simulink model "Quad_Nonlinear_LQR"  (R2020a)
settings: Solver=ode4  StartTime=0.0  StopTime=10.0  FixedStep=.02  RelTol=1e-3
InitFcn:
  | init
undefined symbols (not defined in the file or in its folder): b, d_cg, g, h_cg, J_yy, m2, m_tot, magnitude, miu_k, q1, q2, r_y
settings Model: Creator=Ali  LastModifiedBy=Ali

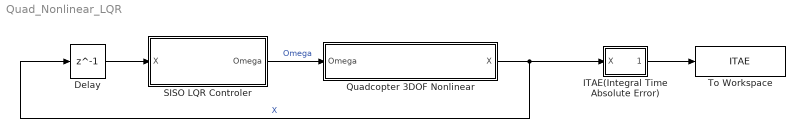
== system Quad_Nonlinear_LQR ==
  Delay : Delay  DelayLength=1
  ITAE(Integral Time Absolute Error) : Subsystem
  Quadcopter 3DOF Nonlinear : Subsystem  TreatAsAtomicUnit=on
  SISO LQR Controler : Subsystem
  To Workspace : ToWorkspace  VariableName=ITAE  SaveFormat=Timeseries  SampleTime=-1
  wires:
  SISO LQR Controler/1(Omega) -> Quadcopter 3DOF Nonlinear/1(Omega)  "Omega"
  Delay/1 -> SISO LQR Controler/1(X)
  Quadcopter 3DOF Nonlinear/1(X) -> ITAE(Integral Time Absolute Error)/1(X), Delay/1  "X"
  ITAE(Integral Time Absolute Error)/1(ITAE) -> To Workspace/1

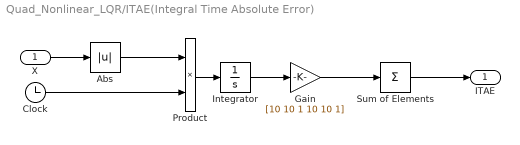
== system Quad_Nonlinear_LQR/ITAE(Integral Time Absolute Error) ==
  X : Inport
  Abs : Abs
  Clock : Clock
  Gain : Gain  Gain=[10 10 1 10 10 1]
  Integrator : Integrator
  Product : Product
  Sum of Elements : Sum  Inputs=+
  ITAE : Outport
  wires:
  Product/1 -> Integrator/1
  Integrator/1 -> Gain/1
  Clock/1 -> Product/2
  Sum of Elements/1 -> ITAE/1
  Abs/1 -> Product/1
  X/1 -> Abs/1
  Gain/1 -> Sum of Elements/1

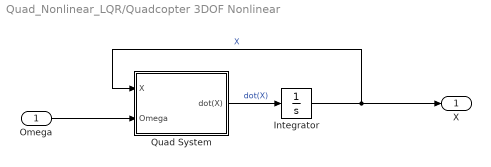
== system Quad_Nonlinear_LQR/Quadcopter 3DOF Nonlinear ==
  Omega : Inport
  Integrator : Integrator  InitialCondition=[-40*pi/180 4*pi/180]
  Quad System : Subsystem
  X : Outport
  wires:
  Integrator/1 -> Quad System/1(X), X/1  "X"
  Quad System/1(dot(X)) -> Integrator/1  "dot(X)"
  Omega/1 -> Quad System/2(Omega)

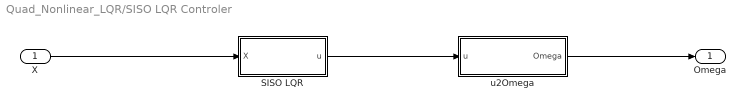
== system Quad_Nonlinear_LQR/SISO LQR Controler ==
  X : Inport
  SISO LQR : Subsystem
  u2Omega : Subsystem
  Omega : Outport
  wires:
  X/1 -> SISO LQR/1(X)
  SISO LQR/1(u) -> u2Omega/1(u)
  u2Omega/1(Omega) -> Omega/1

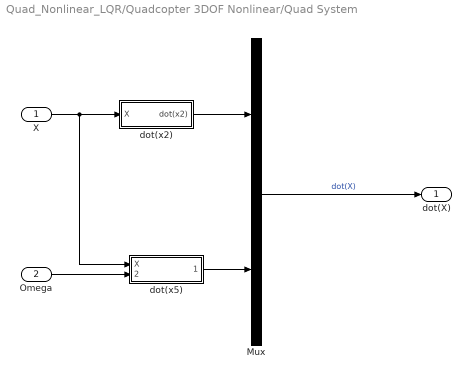
== system Quad_Nonlinear_LQR/Quadcopter 3DOF Nonlinear/Quad System ==
  X : Inport
  Omega : Inport  Port=2
  Mux : Mux  Inputs=2
  dot(x2) : Subsystem
  dot(x5) : Subsystem
  dot(X) : Outport
  wires:
  Mux/1 -> dot(X)/1  "dot(X)"
  dot(x2)/1(dot(x2)) -> Mux/1
  dot(x5)/1(dot(x5)) -> Mux/2
  X/1 -> dot(x5)/1(X), dot(x2)/1(X)
  Omega/1 -> dot(x5)/2(Omega)

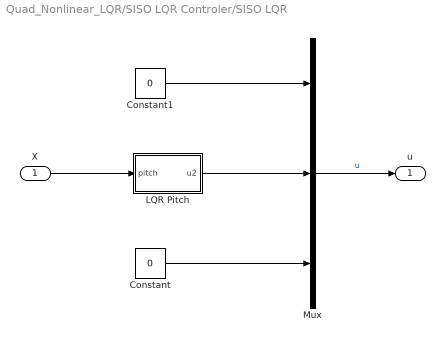
== system Quad_Nonlinear_LQR/SISO LQR Controler/SISO LQR ==
  X : Inport
  Constant : Constant  Value=0
  Constant1 : Constant  Value=0
  LQR Pitch : Subsystem
  Mux : Mux  Inputs=3
  u : Outport
  wires:
  Mux/1 -> u/1  "u"
  Constant1/1 -> Mux/1
  Constant/1 -> Mux/3
  X/1 -> LQR Pitch/1(pitch)
  LQR Pitch/1(u2) -> Mux/2

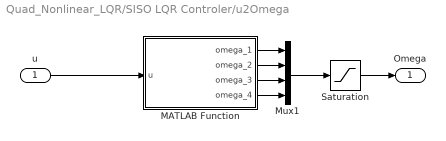
== system Quad_Nonlinear_LQR/SISO LQR Controler/u2Omega ==
  u : Inport
  MATLAB Function : MATLAB Function  TreatAsAtomicUnit=on
  Mux1 : Mux
  Saturation : Saturate  UpperLimit=6000/60*2*pi  LowerLimit=1500/60*2*pi
  Omega : Outport
  wires:
  u/1 -> MATLAB Function/1(u)
  MATLAB Function/3(omega_3) -> Mux1/3
  Mux1/1 -> Saturation/1
  MATLAB Function/1(omega_1) -> Mux1/1
  MATLAB Function/2(omega_2) -> Mux1/2
  MATLAB Function/4(omega_4) -> Mux1/4
  Saturation/1 -> Omega/1

== system Quad_Nonlinear_LQR/Quadcopter 3DOF Nonlinear/Quad System/dot(x2) ==
  X : Inport
  1 : Subsystem
  dot(x2) : Outport
  wires:
  X/1 -> 1/1(X)  "X"
  1/1(x5cos(x1)) -> dot(x2)/1

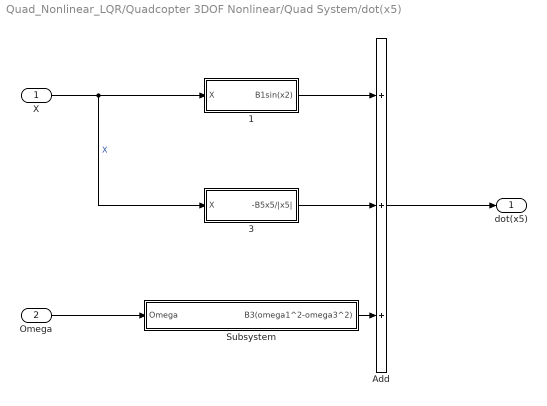
== system Quad_Nonlinear_LQR/Quadcopter 3DOF Nonlinear/Quad System/dot(x5) ==
  X : Inport
  Omega : Inport  Port=2
  1 : Subsystem
  3 : Subsystem
  Add : Sum  Inputs=+++
  Subsystem : Subsystem
  dot(x5) : Outport
  wires:
  X/1 -> 3/1(X), 1/1(X)  "X"
  Omega/1 -> Subsystem/1(Omega)
  Add/1 -> dot(x5)/1
  Subsystem/1(B3(omega1^2-omega3^2)) -> Add/3
  3/1("-B5x5/|x5| ") -> Add/2
  1/1(B1sin(x2)) -> Add/1

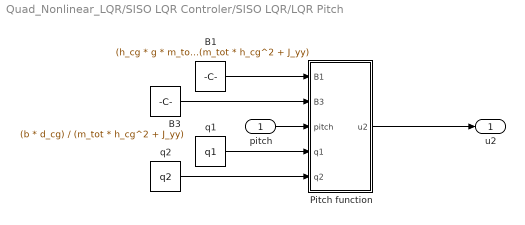
== system Quad_Nonlinear_LQR/SISO LQR Controler/SISO LQR/LQR Pitch ==
  pitch : Inport
  B1 : Constant  Value=(h_cg * g * m_tot) / (m_tot * h_cg^2 + J_yy)
  B3 : Constant  Value=(b * d_cg) / (m_tot * h_cg^2 + J_yy)
  Pitch function : MATLAB Function  TreatAsAtomicUnit=on
  q1 : Constant  Value=q1
  q2 : Constant  Value=q2
  u2 : Outport
  wires:
  Pitch function/1(u2) -> u2/1
  pitch/1 -> Pitch function/3(pitch)
  B1/1 -> Pitch function/1(B1)
  B3/1 -> Pitch function/2(B3)
  q1/1 -> Pitch function/4(q1)
  q2/1 -> Pitch function/5(q2)

== system Quad_Nonlinear_LQR/Quadcopter 3DOF Nonlinear/Quad System/dot(x2)/1 ==
  X : Inport
  Selector : Selector  InputPortWidth=2  IndexOptions=Index vector (dialog)  Indices=[2]  OutputSizes=1
  x5cos(x1) : Outport
  wires:
  X/1 -> Selector/1  "x"
  Selector/1 -> x5cos(x1)/1

== system Quad_Nonlinear_LQR/Quadcopter 3DOF Nonlinear/Quad System/dot(x5)/1 ==
  X : Inport
  Selector : Selector  InputPortWidth=2  IndexOptions=Index vector (dialog)  Indices=[1]  OutputSizes=1
  Subsystem : Subsystem
  B1sin(x2) : Outport
  wires:
  X/1 -> Selector/1  "x"
  Subsystem/1(B1sin(x2)) -> B1sin(x2)/1
  Selector/1 -> Subsystem/1(x2)

== system Quad_Nonlinear_LQR/Quadcopter 3DOF Nonlinear/Quad System/dot(x5)/3 ==
  X : Inport
  Selector : Selector  InputPortWidth=2  IndexOptions=Index vector (dialog)  Indices=[2]  OutputSizes=1
  Subsystem : Subsystem
  "-B5x5/|x5| " : Outport
  wires:
  X/1 -> Selector/1  "x"
  Subsystem/1("-B5x5/|x5| ") -> "-B5x5/|x5| "/1
  Selector/1 -> Subsystem/1(x5)

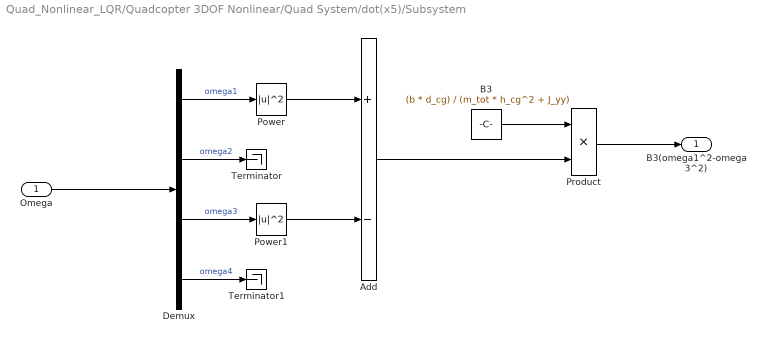
== system Quad_Nonlinear_LQR/Quadcopter 3DOF Nonlinear/Quad System/dot(x5)/Subsystem ==
  Omega : Inport
  Add : Sum  Inputs=+-
  B3 : Constant  Value=(b * d_cg) / (m_tot * h_cg^2 + J_yy)
  Demux : Demux
  Power : Math  Operator=magnitude^2  SaturateOnIntegerOverflow=on
  Power1 : Math  Operator=magnitude^2  SaturateOnIntegerOverflow=on
  Product : Product
  Terminator : Terminator
  Terminator1 : Terminator
  B3(omega1^2-omega3^2) : Outport
  wires:
  Product/1 -> B3(omega1^2-omega3^2)/1
  Power1/1 -> Add/2
  Add/1 -> Product/2
  Power/1 -> Add/1
  B3/1 -> Product/1
  Omega/1 -> Demux/1
  Demux/3 -> Power1/1  "omega3"
  Demux/1 -> Power/1  "omega1"
  Demux/2 -> Terminator/1  "omega2"
  Demux/4 -> Terminator1/1  "omega4"

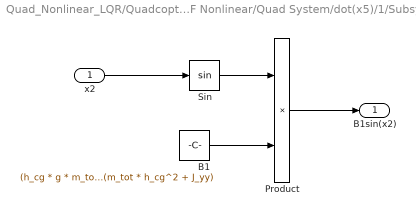
== system Quad_Nonlinear_LQR/Quadcopter 3DOF Nonlinear/Quad System/dot(x5)/1/Subsystem ==
  x2 : Inport
  B1 : Constant  Value=(h_cg * g * m_tot) / (m_tot * h_cg^2 + J_yy)
  Product : Product
  Sin : Trigonometry
  B1sin(x2) : Outport
  wires:
  Product/1 -> B1sin(x2)/1
  x2/1 -> Sin/1
  Sin/1 -> Product/1
  B1/1 -> Product/2

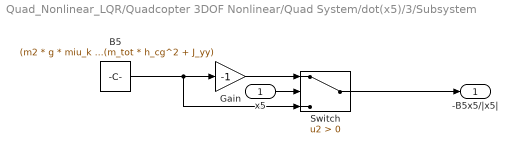
== system Quad_Nonlinear_LQR/Quadcopter 3DOF Nonlinear/Quad System/dot(x5)/3/Subsystem ==
  x5 : Inport
  B5 : Constant  Value=(m2 * g * miu_k * r_y) / (m_tot * h_cg^2 + J_yy)
  Gain : Gain  Gain=-1
  Switch : Switch  Criteria=u2 > Threshold
  "-B5x5/|x5| " : Outport
  wires:
  Switch/1 -> "-B5x5/|x5| "/1
  B5/1 -> Switch/3, Gain/1
  x5/1 -> Switch/2
  Gain/1 -> Switch/1

== matlab function Quad_Nonlinear_LQR/SISO LQR Controler/SISO LQR/LQR Pitch/Pitch function ==
  data: B1 input; B3 input; pitch input; u2 output; q1 input; q2 input
function u2  = fcn(B1, B3, pitch, q1, q2)

x2     = pitch(1);
A22    = 0; %da2dx2
A25    = 1; %da2dx5
A52    = B1 * cos(x2); %da5dx2
A55    = 0; %da5dx5

A      = [A22, A25 ;
          A52, A55];
B      = [0  ;
          B3];
a      = A(2);
b      = B(2);

R      = 1;
R_inv  = R^-1;
K_ans = zeros(2, 2);
% algebraic_riccati = K * A + A' * K - K * B * R^-1 * B' * K + Q;
% first equation q1 + 2*a*k12 - (b^2*k12^2)/R = 0
% Ans1 K12 = -m*(k + (k^2 + Q11)^(1/2))
% Ans2 K12 = -m*(k - (k^2 + Q11)^(1/2))
K12 = zeros(1, 2);
K12(1) = (R*(a + ((R*a^2 + q1*b^2)/R)^(1/2)))/b^2;
K12(2) = (R*(a - ((R*a^2 + q1*b^2)/R)^(1/2)))/b^2;
stable = false; % check stability answer for break code
for i = 1:length(K12)
    % Second equation 2*k12 + q2 - (b^2*k22^2)/R = 0
    % Ans1 K12 =  (2*k12 + q2)^(1/2)/(R^(1/2)*b)
    % Ans2 K12 = -(2*k12 + q2)^(1/2)/(R^(1/2)*b)
    valid22 = [true; true]; % for validation in complex number
    K22 = zeros(1, 2);
    if (2*K12(i) + q2) < 0
        valid22(i) = false;
    end
    if valid22(i)
        K22(1) =  (R^(1/2)*(2*K12(i) + q2)^(1/2))/b;
        K22(2) = -(R^(1/2)*(2*K12(i) + q2)^(1/2))/b;
    else
        continue;
    end
    for j = 1:length(K22)
        % Last equation k11 + a*k22 - (b^2*k12*k22)/R = 0
        % Ans R*k12*k22*b^2 - a*k22
        K11 = (K12(i)*K22(j)*b^2)/R - a*K22(j);
        temp_K = zeros(2, 2);
        temp_K(1, 1) = K11;
        temp_K(1, 2) = K12(i);
        temp_K(2, 1) = K12(i);
        temp_K(2, 2) = K22(j);
        if all(eig(A - B * R^(-1)* B' * temp_K) < 0)
            K_ans = temp_K;
            stable = true;
            break;
        end
    end
    if stable
        break;
    end
end

u2 = -R_inv*B'*K_ans*pitch;

== matlab function Quad_Nonlinear_LQR/SISO LQR Controler/u2Omega/MATLAB Function ==
  data: u input size=3; omega_1 output size=1; omega_2 output size=1; omega_3 output size=1; omega_4 output size=1
function [omega_1, omega_2, omega_3, omega_4] = fcn(u)
u1 = u(1);
u2 = u(2);
u3 = u(3);
% control effort
u4 = ones(1, length(u1)) * 4 * rpm2rad_sec(2000)^2;
% calculate omega
if (u4 + u3 + 2 * u2) / 4 > 0
    omega_1 = sqrt((u4 + u3 + 2 * u2) / 4);
else
    omega_1 = 0;
end
if (u4 + u3 - 2 * u2) / 4 > 0
    omega_3 = sqrt((u4 + u3 - 2 * u2) / 4);
else
    omega_3 = 0;
end
if (u4 - u3 + 2 * u1) / 4 > 0
    omega_2 = sqrt((u4 - u3 + 2 * u1) / 4);
else
    omega_2 = 0;
end
if (u4 - u3 - 2 * u1) / 4 > 0
    omega_4 = sqrt((u4 - u3 - 2 * u1) / 4);
else
    omega_4 = 0;
end
end
%% functions
% rpm to rad/sec
function rad = rpm2rad_sec(rpm)
rad = rpm / 60 * 2 * pi;
end
